simulink model "inverter"  (R2024b)
settings: Solver=VariableStepAuto  StartTime=0.0  StopTime=3  RelTol=1e-3
values from neighbouring files (symbols this model uses):
  pmsm =     [foc.mat]    (also in inverter.mat; speed_control.mat; vbyf.mat)
  Ts = 2.5e-05    [foc.mat]    (also in inverter.mat; speed_control.mat; vbyf.mat)
libraries: mcbplantlib x1, autolibpmsminterior x1
settings Model: Creator=realf  LastModifiedBy=realf

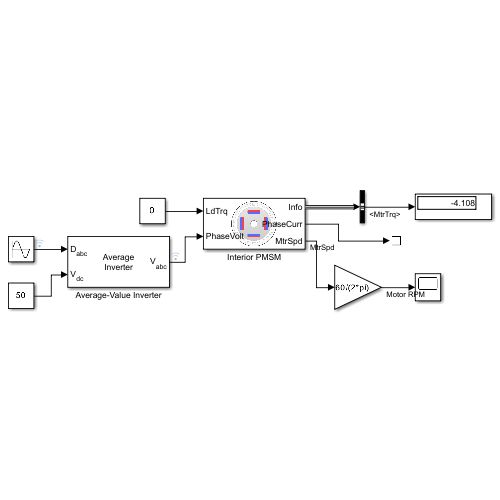
[thumbnail: Simulink's stored preview of the top-level diagram]
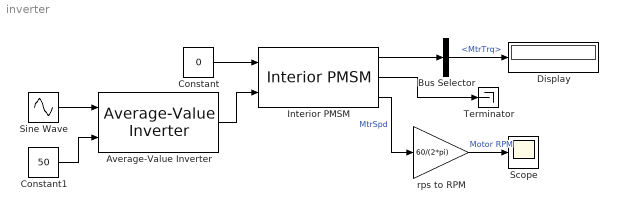
== system inverter ==
  Average-Value Inverter : mcbplantlib/Average-Value Inverter
      settings: LibrarySourceBlock=mcblib/Electrical Systems/Inverters/Average-Value Inverter
  Bus Selector : BusSelector  OutputSignals=MtrTrq
  Constant : Constant  Value=0
  Constant1 : Constant  Value=50
  Display : Display
  Interior PMSM : autolibpmsminterior/Interior PMSM  port_config=Torque  sim_type=Discrete  Ts=Ts  P=pmsm.p  Rs=pmsm.Rs  Ldq=[pmsm.Ld, pmsm.Lq]  KConstText=Permanent flux linkage constant (lambda_pm):  lambda_pm=pmsm.FluxPM  Ke=159.9771  mechanical=[pmsm.J, 0, 0]  idq0=[0 0]  theta_init=0  omega_init=0  KConst=pmsm.FluxPM  lambda_pm_calc=pmsm.FluxPM  Kt=0.07  RefBlkName='autolibpmsminterior/Interior PMSM'  aMode=5
      settings: LibrarySourceBlock=mcblib/Electrical Systems/Motors/Interior PMSM
  Scope : Scope
  Sine Wave : Sin  Bias=0.5  Frequency=30  Phase=[0, -2*pi/3, -4*pi/3]  SampleTime=0
  Terminator : Terminator
  rps to RPM : Gain  Gain=60/(2*pi)
  wires:
  Sine Wave/1 -> Average-Value Inverter/1
  Interior PMSM/3 -> rps to RPM/1  "MtrSpd"
  Constant1/1 -> Average-Value Inverter/2
  Average-Value Inverter/1 -> Interior PMSM/2
  Constant/1 -> Interior PMSM/1
  Interior PMSM/1 -> Bus Selector/1
  Interior PMSM/2 -> Terminator/1
  Bus Selector/1 -> Display/1  "<MtrTrq>"
  rps to RPM/1 -> Scope/1  "Motor RPM"
